simulink model "opid"  (Simulink 7.3)
settings: Solver=ode45  StartTime=0.0  StopTime=1200  RelTol=1e-3
values from neighbouring files (symbols this model uses):
  D = 0    [MagnetLev.m]
undefined symbols (not defined in the file or in its folder): I, P
settings Model: Creator=Administrator  LastModifiedBy=sn00632
settings DataIOCC: LimitDataPoints=off
settings OptimizationCC: InlineInvariantSignals=on  InitFltsAndDblsToZero=on
settings DebuggingCC: SaveWithParameterizedLinksMsg=none  SignalResolutionControl=TryResolveAllWithWarning  SolverPrmCheckMsg=none  MultiTaskDSMMsg=warning  MultiTaskCondExecSysMsg=none  StrictBusMsg=None
settings RTWCC: IncludeERTFirstTime=on
settings GRTTargetCC: TargetFcnLib=ansi_tfl_tmw.mat

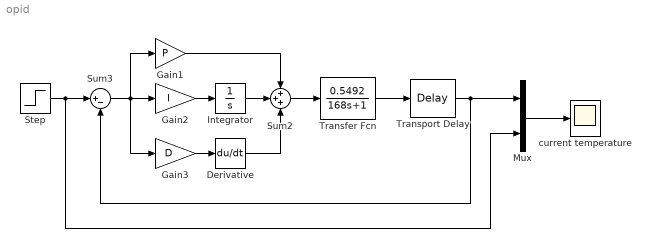
== system opid ==
  Derivative : Derivative
  Gain1 : Gain  Gain=P  ParameterDataType=sfix(16)  ParameterScaling=2^0  OutDataType=sfix(16)  OutScaling=2^0
  Gain2 : Gain  Gain=I  ParameterDataType=sfix(16)  ParameterScaling=2^0  OutDataType=sfix(16)  OutScaling=2^0
  Gain3 : Gain  Gain=D  ParameterDataType=sfix(16)  ParameterScaling=2^0  OutDataType=sfix(16)  OutScaling=2^0
  Integrator : Integrator
  Mux : Mux  Inputs=2
  Step : Step  Time=0  After=80  SampleTime=0
  Sum2 : Sum  Inputs=+++  OutDataType=sfix(16)  OutScaling=2^0
  Sum3 : Sum  Inputs=|+-  OutDataType=sfix(16)  OutScaling=2^0
  Transfer Fcn : TransferFcn  Numerator=[0.5492]  Denominator=[168 1]
  Transport Delay : TransportDelay  DelayTime=58.5
  current temperature : Scope
      settings: TimeRange=1200  YMin=0  YMax=20  SaveName=ScopeData2
  wires:
  Transport Delay/1 -> Sum3/2, Mux/1
  Sum2/1 -> Transfer Fcn/1
  Gain3/1 -> Derivative/1
  Gain2/1 -> Integrator/1
  Integrator/1 -> Sum2/2
  Derivative/1 -> Sum2/3
  Gain1/1 -> Sum2/1
  Sum3/1 -> Gain1/1, Gain3/1, Gain2/1
  Transfer Fcn/1 -> Transport Delay/1
  Step/1 -> Sum3/1, Mux/2
  Mux/1 -> current temperature/1
